simulink model "HFV_model"  (R2019b)
settings: Solver=VariableStepAuto  StartTime=0.0  StopTime=20  FixedStep=0.1  RelTol=1e-3
libraries: simulink_extras x2, simulink x1
settings Model: Creator=114-AO  LastModifiedBy=114-AO

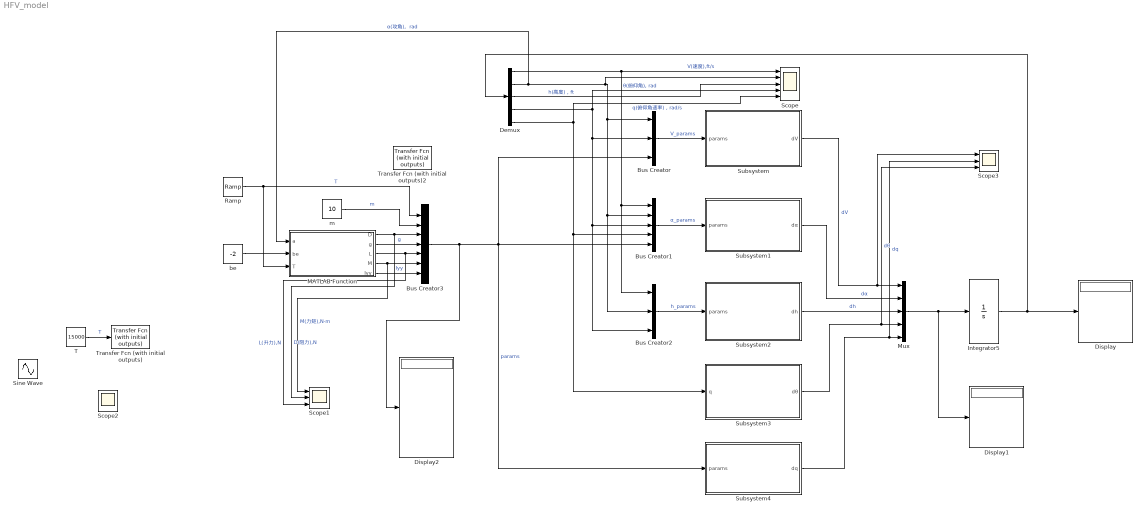
== system HFV_model ==
  Bus Creator : BusCreator  Inputs=3
  Bus Creator1 : BusCreator  Inputs=5
  Bus Creator2 : BusCreator  Inputs=3
  Bus Creator3 : BusCreator  Inputs=7
  Demux : Demux  Outputs=5
  Display : Display
  Display1 : Display
  Display2 : Display
  Integrator5 : Integrator  InitialCondition=eps
  MATLAB Function : MATLAB Function  TreatAsAtomicUnit=on
  Mux : Mux  Inputs=5
  Ramp : simulink/Sources/Ramp  slope=100  start=0  InitialOutput=10000
  Scope : Scope  NumInputPorts=5
  Scope1 : Scope  NumInputPorts=3
  Scope2 : Scope  NumInputPorts=3
  Scope3 : Scope  NumInputPorts=3
  Sine Wave : Sin  Amplitude=2500  Bias=15000  Frequency=0.5  SampleTime=0
  Subsystem : Subsystem
  Subsystem1 : Subsystem
  Subsystem2 : Subsystem
  Subsystem3 : Subsystem
  Subsystem4 : Subsystem
  T : Constant  Value=15000
  Transfer Fcn (with initial outputs) : simulink_extras/Additional Linear/Transfer Fcn (with initial outputs)  N=[1]  D="[2  1]"  Y0=10000  U0=0
  Transfer Fcn (with initial outputs)2 : simulink_extras/Additional Linear/Transfer Fcn (with initial outputs)  N=[1]  D="[1  1]"  Y0=30  U0=0
  be : Constant  Value=-2
  m : Constant  Value=10
  wires:
  Subsystem/1(dV) -> Scope3/1, Mux/1  "dV"
  Subsystem2/1(dh) -> Mux/3  "dh"
  Subsystem3/1(dθ) -> Scope3/3, Mux/4  "dθ"
  Subsystem4/1(dq) -> Scope3/2, Mux/5  "dq"
  Integrator5/1 -> Demux/1, Display/1
  Mux/1 -> Display1/1, Integrator5/1
  Subsystem1/1(dα) -> Mux/2  "dα"
  Demux/1 -> Scope/1, Bus Creator2/1, Bus Creator1/1  "V(速度),ft/s"
  Demux/2 -> MATLAB Function/1(a), Scope/2, Bus Creator/1, Bus Creator2/2, Bus Creator1/2  "α(攻角),  rad"
  Demux/4 -> Bus Creator2/3, Bus Creator1/3, Bus Creator/2, Scope/4  "θ(俯仰角), rad"
  Demux/5 -> Subsystem3/1(q), Bus Creator1/4, Scope/5  "q(俯仰角速率)，rad/s"
  Bus Creator/1 -> Subsystem/1(params)  "V_params"
  Bus Creator1/1 -> Subsystem1/1(params)  "α_params"
  Bus Creator2/1 -> Subsystem2/1(params)  "h_params"
  Bus Creator3/1 -> Display2/1, Bus Creator/3, Subsystem4/1(params), Bus Creator1/5  "params"
  MATLAB Function/5(Iyy) -> Bus Creator3/7  "Iyy"
  T/1 -> Transfer Fcn (with initial outputs)/1  "T"
  MATLAB Function/1(D) -> Scope1/2, Bus Creator3/3  "D(阻力),N"
  MATLAB Function/2(g) -> Bus Creator3/4  "g"
  m/1 -> Bus Creator3/2  "m"
  MATLAB Function/3(L) -> Scope1/3, Bus Creator3/5  "L(升力),N"
  MATLAB Function/4(M) -> Scope1/1, Bus Creator3/6  "M(力矩),N·m"
  be/1 -> MATLAB Function/2(be)
  Ramp/1 -> MATLAB Function/3(T), Bus Creator3/1  "T"
  Demux/3 -> Scope/3  "h(高度)，ft"

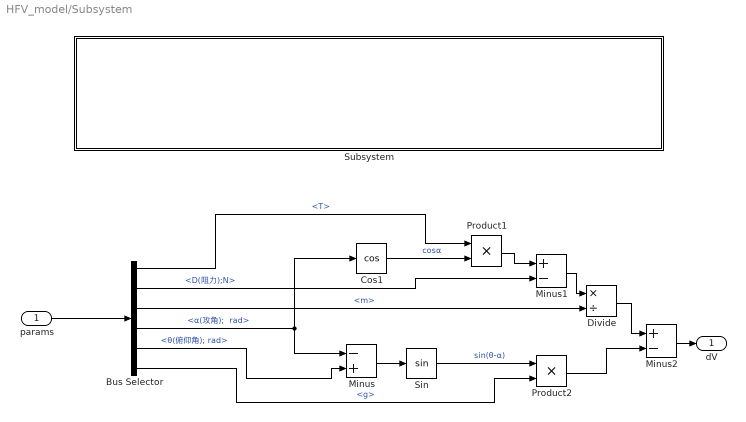
== system HFV_model/Subsystem ==
  params : Inport
  Bus Selector : BusSelector  OutputSignals="params.T,params.D(阻力);N,params.m,α(攻角);  rad,θ(俯仰角); rad,params.g"
  Cos1 : Trigonometry  Operator=cos
  Divide : Product  Inputs=*/
  Minus : Sum  Inputs=-+
  Minus1 : Sum  Inputs=+-
  Minus2 : Sum  Inputs=+-
  Product1 : Product
  Product2 : Product
  Sin : Trigonometry
  Subsystem : Subsystem
      mask Display: image('E:\desktop\TBCC1\images\V_.jpg'); % Use "Edit Image" on toolstrip to change.
  dV : Outport
  wires:
  Product1/1 -> Minus1/1
  Bus Selector/4 -> Minus/1, Cos1/1  "<α(攻角);  rad>"
  Bus Selector/5 -> Minus/2  "<θ(俯仰角); rad>"
  Minus2/1 -> dV/1
  Sin/1 -> Product2/1  "sin(θ-α)"
  Divide/1 -> Minus2/1
  Product2/1 -> Minus2/2
  Minus1/1 -> Divide/1
  Cos1/1 -> Product1/2  "cosα"
  Bus Selector/6 -> Product2/2  "<g>"
  Bus Selector/3 -> Divide/2  "<m>"
  Bus Selector/2 -> Minus1/2  "<D(阻力);N>"
  Minus/1 -> Sin/1
  params/1 -> Bus Selector/1
  Bus Selector/1 -> Product1/1  "<T>"

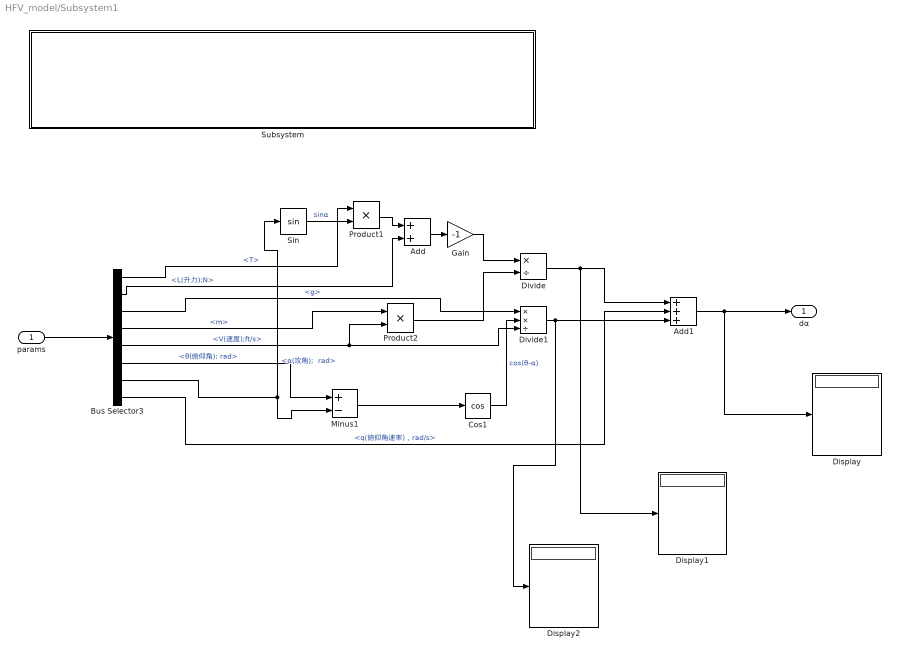
== system HFV_model/Subsystem1 ==
  params : Inport
  Add : Sum
  Add1 : Sum  Inputs=+++
  Bus Selector3 : BusSelector  OutputSignals="params.T,params.L(升力);N,params.g,params.m,V(速度);ft/s,θ(俯仰角); rad,α(攻角);  rad,q(俯仰角速率)，rad/s"
  Cos1 : Trigonometry  Operator=cos
  Display : Display
  Display1 : Display
  Display2 : Display
  Divide : Product  Inputs=*/
  Divide1 : Product  Inputs=**/
  Gain : Gain  Gain=-1
  Minus1 : Sum  Inputs=+-
  Product1 : Product
  Product2 : Product
  Sin : Trigonometry
  Subsystem : Subsystem
      mask Display: image('E:\desktop\TBCC1\images\a_.jpg'); % Use "Edit Image" on toolstrip to change.
  dα : Outport
  wires:
  Add/1 -> Gain/1
  Product1/1 -> Add/1
  Minus1/1 -> Cos1/1
  Add1/1 -> Display/1, dα/1
  Product2/1 -> Divide/2
  Cos1/1 -> Divide1/2  "cos(θ-α)"
  Sin/1 -> Product1/2  "sinα"
  Divide/1 -> Display1/1, Add1/1
  Divide1/1 -> Display2/1, Add1/3
  Bus Selector3/4 -> Product2/1  "<m>"
  Bus Selector3/3 -> Divide1/1  "<g>"
  Bus Selector3/8 -> Add1/2  "<q(俯仰角速率)，rad/s>"
  Bus Selector3/2 -> Add/2  "<L(升力);N>"
  Bus Selector3/1 -> Product1/1  "<T>"
  Bus Selector3/7 -> Sin/1, Minus1/2  "<α(攻角);  rad>"
  Bus Selector3/6 -> Minus1/1  "<θ(俯仰角); rad>"
  params/1 -> Bus Selector3/1
  Bus Selector3/5 -> Product2/2, Divide1/3  "<V(速度);ft/s>"
  Gain/1 -> Divide/1

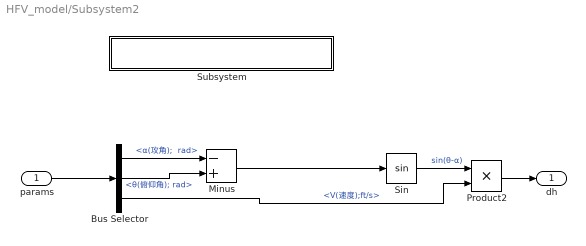
== system HFV_model/Subsystem2 ==
  params : Inport
  Bus Selector : BusSelector  OutputSignals="α(攻角);  rad,θ(俯仰角); rad,V(速度);ft/s"
  Minus : Sum  Inputs=-+
  Product2 : Product
  Sin : Trigonometry
  Subsystem : Subsystem
      mask Display: image('E:\desktop\TBCC1\images\h_.jpg'); % Use "Edit Image" on toolstrip to change.
  dh : Outport
  wires:
  Sin/1 -> Product2/1  "sin(θ-α)"
  Bus Selector/1 -> Minus/1  "<α(攻角);  rad>"
  Product2/1 -> dh/1
  Bus Selector/2 -> Minus/2  "<θ(俯仰角); rad>"
  Bus Selector/3 -> Product2/2  "<V(速度);ft/s>"
  params/1 -> Bus Selector/1
  Minus/1 -> Sin/1

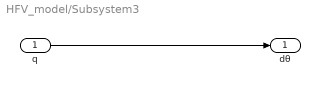
== system HFV_model/Subsystem3 ==
  q : Inport
  dθ : Outport
  wires:
  q/1 -> dθ/1

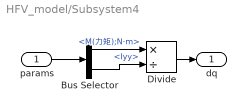
== system HFV_model/Subsystem4 ==
  params : Inport
  Bus Selector : BusSelector  OutputSignals=M(力矩);N·m,Iyy
  Divide : Product  Inputs=*/
  dq : Outport
  wires:
  Bus Selector/1 -> Divide/1  "<M(力矩);N·m>"
  Divide/1 -> dq/1
  Bus Selector/2 -> Divide/2  "<Iyy>"
  params/1 -> Bus Selector/1

== system HFV_model/Subsystem/Subsystem ==

== system HFV_model/Subsystem1/Subsystem ==

== system HFV_model/Subsystem2/Subsystem ==

== matlab function HFV_model/MATLAB Function ==
  data: D output; g output; a input; L output; be input; M output; Iyy output; T input
function [D, g, L, M, Iyy] = HFV_Params(a, be, T)

m = 30;
g = 32.17;
Iyy = 500000;
S = 17;
p0 = 6.7429*10^(-5);
hs = 21358.8;
h0 = 85000;
c_ = 17;
zT = 8.36;
ce = -1.2897;
q_ = 70;

C0L = -0.018714;
CaL = 4.6773;
CbeL = 0.76224;
C0D = 0.010131;
CaD = -0.045315;
Ca2D = 5.8224;
CbeD = 2.7699*0.0001;
Cbe2D = 0.81993;
C0Ma = -0.18979;
CaMa = 2.1335;
Ca2Ma = 6.2926;

% b1 = -3.7693*10^5;
% b2 = -3.7225*10^4;
% b3 = 2.6814*10^4;
% b4 = -1.7277*10^4;
% b5 = 3.5542*10^4;
% b6 = -2.4216*10^3;
% b7 = 6.3785*10^3;
% b8 = -1.0090*10^2;


L = q_*S*(CaL*a + CbeL*be + C0L);
D = q_*S*(Ca2D*a^2 + CaD*a +Cbe2D*be^2 + CbeD*be + C0D);
M = q_*S*c_*(Ca2Ma*a^2 + CaMa*a + C0Ma+ce*be);% M = 1;
% M = zT*T + q_*S*c_*(Ca2Ma*a^2 + CaMa*a + C0Ma+ce*be);% M = 1;

end
